simulink model "Receive_Ethernet_UDP"  (R2024a)
settings: Solver=ode4  StartTime=0.0  StopTime=inf  FixedStep=0.01  RelTol=1e-3
undefined symbols (not defined in the file or in its folder): f, gray
libraries: sldrtlib x1, instrumentlib x1
settings Model: Creator=hyeon-yongjeong  LastModifiedBy=LG gram 17 - HW dev

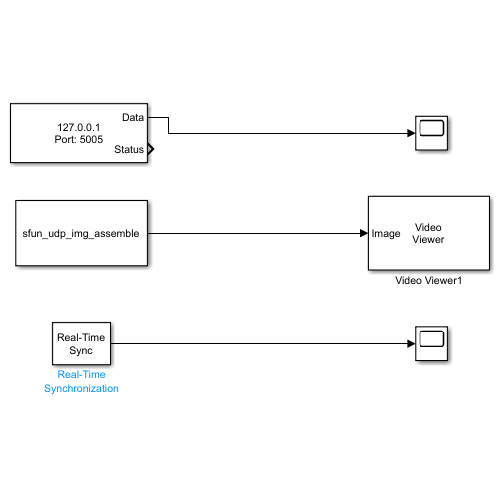
[thumbnail: Simulink's stored preview of the top-level diagram]
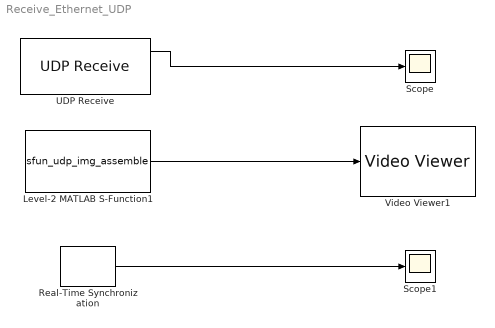
== system Receive_Ethernet_UDP ==
  Level-2 MATLAB S-Function1 : M-S-Function  FunctionName=sfun_udp_img_assemble  Parameters=5006, [240 320], 8192, 0.1
  Real-Time Synchronization : sldrtlib/Real-Time Synchronization  SampleTime=0.01  MaxMissedTicks=inf  ShowMissedTicks=on  YieldWhenWaiting=off
  Scope : Scope
  Scope1 : Scope
  UDP Receive : instrumentlib/UDP Receive  LocalAddress=127.0.0.1  LocalPort=5005  EnablePortSharing=off  Host=0.0.0.0  Port=5005  GetLatestData=off  DataSize=[6 1]  DataType=single  ASCIIFormatting=%f,  Terminator=LF  CustomTerminator=10  ByteOrder=little-endian  EnableBlockingMode=off  Timeout=10  SampleTime=0.01  SimulateUsing=Interpreted execution
  Video Viewer1 : VideoViewer  colormapValue=gray(256)  FigPos=[177 1229.33333333333 652 454]
  wires:
  UDP Receive/1 -> Scope/1
  Level-2 MATLAB S-Function1/1 -> Video Viewer1/1
  Real-Time Synchronization/1 -> Scope1/1
